simulink model "Product_TestGen4"  (R2017b)
settings: Solver=FixedStepDiscrete  StartTime=0.0  StopTime=10.0  RelTol=1e-3
undefined symbols (not defined in the file): Block_TestLib, enable_trigger
settings Model: Creator=ktrinh  LastModifiedBy=ktrinh
settings DebuggingCC: ParameterOverflowMsg=none

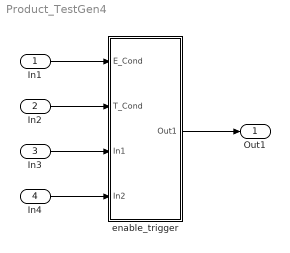
== system Product_TestGen4 ==
  In1 : Inport
  In2 : Inport  Port=2
  In3 : Inport  Port=3
  In4 : Inport  Port=4
  enable_trigger : Subsystem  AncestorBlock=Block_TestLib/enable_trigger
  Out1 : Outport
  wires:
  In1/1 -> enable_trigger/1(E_Cond)
  In2/1 -> enable_trigger/2(T_Cond)
  In3/1 -> enable_trigger/3(In1)
  In4/1 -> enable_trigger/4(In2)
  enable_trigger/1(Out1) -> Out1/1

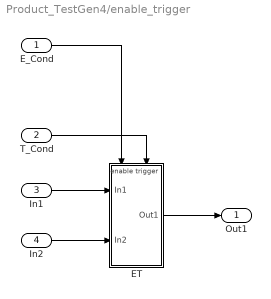
== system Product_TestGen4/enable_trigger ==
  E_Cond : Inport  OutDataTypeStr=boolean
  T_Cond : Inport  Port=2  OutDataTypeStr=boolean
  In1 : Inport  Port=3
  In2 : Inport  Port=4
  ET : Subsystem  TreatAsAtomicUnit=on
  Out1 : Outport
  wires:
  T_Cond/1 -> ET/Trigger
  E_Cond/1 -> ET/Enable
  In1/1 -> ET/1(In1)
  In2/1 -> ET/2(In2)
  ET/1(Out1) -> Out1/1

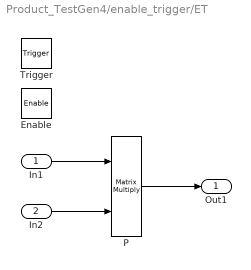
== system Product_TestGen4/enable_trigger/ET ==
  In1 : Inport  OutDataTypeStr=uint8  PortDimensions=1
  In2 : Inport  Port=2  OutDataTypeStr=uint8  PortDimensions=1
  Enable : EnablePort
  Trigger : TriggerPort  VariantControl=Variant
  P : Product  Multiplication=Matrix(*)  OutDataTypeStr=uint8  InputSameDT=on
  Out1 : Outport
  wires:
  In1/1 -> P/1
  In2/1 -> P/2
  P/1 -> Out1/1
